simulink model "suspensionMBD_2"  (R2020b)
settings: Solver=VariableStepAuto  StartTime=0.0  StopTime=100  RelTol=1e-3
undefined symbols (not defined in the file): b, k1, k2, m1, m2
settings Model: Creator=DELL  LastModifiedBy=DELL
settings DataIOCC: ExternalInput=[t stin]  LoadExternalInput=on

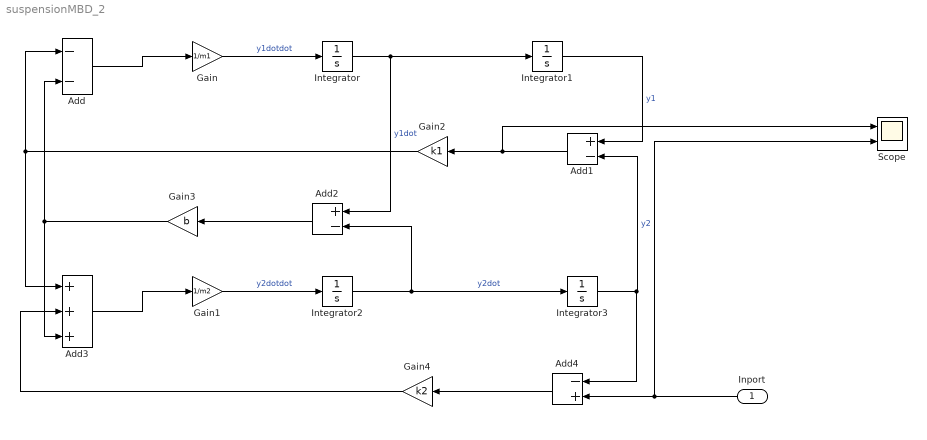
== system suspensionMBD_2 ==
  Inport : Inport
  Add : Sum  Inputs=--
  Add1 : Sum  Inputs=+-
  Add2 : Sum  Inputs=+-
  Add3 : Sum  Inputs=+++
  Add4 : Sum  Inputs=-+
  Gain : Gain  Gain=1/m1
  Gain1 : Gain  Gain=1/m2
  Gain2 : Gain  Gain=k1
  Gain3 : Gain  Gain=b
  Gain4 : Gain  Gain=k2
  Integrator{,1..3} (4 alike) : Integrator
  Scope : Scope  NumInputPorts=2
  wires:
  Integrator/1 -> Add2/1, Integrator1/1  "y1dot"
  Integrator1/1 -> Add1/1  "y1"
  Gain/1 -> Integrator/1  "y1dotdot"
  Integrator2/1 -> Add2/2, Integrator3/1  "y2dot"
  Gain1/1 -> Integrator2/1  "y2dotdot"
  Integrator3/1 -> Add4/1, Add1/2  "y2"
  Add/1 -> Gain/1
  Add1/1 -> Scope/1, Gain2/1
  Gain3/1 -> Add3/3, Add/2
  Add2/1 -> Gain3/1
  Add3/1 -> Gain1/1
  Add4/1 -> Gain4/1
  Gain2/1 -> Add3/1, Add/1
  Gain4/1 -> Add3/2
  Inport/1 -> Scope/2, Add4/2
